simulink model "Robot_control"  (Simulink 8.0)
settings: Solver=ode45  SolverMode=SingleTasking  StartTime=0.0  StopTime=10  RelTol=1e-3
libraries: mblibv1 x4, vrlib x1
settings Model: Creator=zigg  LastModifiedBy=nakano  CovMetricSettings=dwe  CovHtmlReporting=off  covSaveCumulativeToWorkspaceVar=off  CovSaveSingleToWorkspaceVar=off  CovExternalEMLEnable=on
settings DataIOCC: LimitDataPoints=off  SaveFormat=StructureWithTime
settings OptimizationCC: ExpressionDepthLimit=128
settings DebuggingCC: UnderspecifiedInitializationDetection=Simplified  MergeDetectMultiDrivingBlocksExec=error  SolverPrmCheckMsg=none  FcnCallInpInsideContextMsg=EnableAllAsWarning  FrameProcessingCompatibilityMsg=error  StateNameClashWarn=none  SFUnexpectedBacktrackingDiag=error  SFNoUnconditionalDefaultTransitionDiag=error
settings HardwareCC: ProdBitPerPointer=64  ProdLargestAtomicFloat=Float  ProdIntDivRoundTo=Zero  ProdEndianess=LittleEndian  ProdHWDeviceType=Specified
settings ModelReferenceCC: PropagateSignalLabelsOutOfModel=on
settings CodeAppCC: CustomSymbolStrType=$N$R$M_T
settings GRTTargetCC: CodeReplacementLibrary=C99 (ISO)  GeneratePreprocessorConditionals=Use local settings

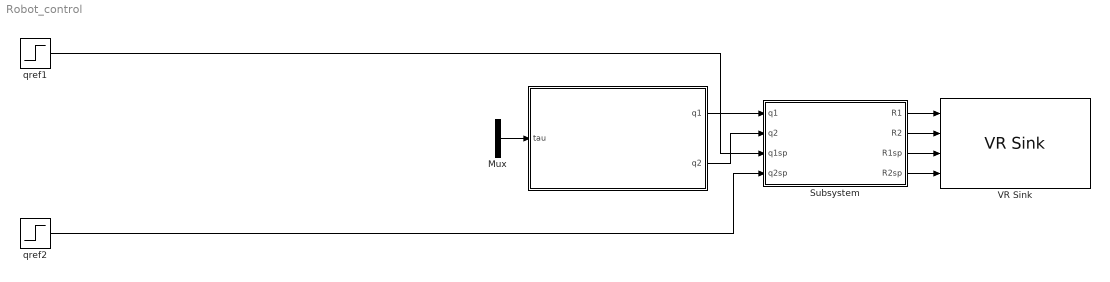
== system Robot_control ==
  "  " : Subsystem
  Mux : Mux  Inputs=2
  Subsystem : Subsystem
  VR Sink : vrlib/VR Sink  InstantiateOnLoad=on  SampleTime=0.1  ViewEnable=on  RemoteChange=off  RemoteView=off  FieldsWritten=Joint1.rotation.4.1.1.double#Joint2.rotation.4.1.1.double#Joint1_SP.rotation.4.1.1.double#Joint2_SP.rotation.4.1.1.double  WorldFileName=my_robot.wrl  AutoView=off  VideoDimensions=[]  AllowVariableSize=off
  qref1 : Step  SampleTime=0
  qref2 : Step  SampleTime=0
  wires:
  Subsystem/1(R1) -> VR Sink/1
  Subsystem/2(R2) -> VR Sink/2
  Subsystem/3(R1sp) -> VR Sink/3
  Subsystem/4(R2sp) -> VR Sink/4
  "  "/1(q1) -> Subsystem/1(q1)
  "  "/2(q2) -> Subsystem/2(q2)
  qref2/1 -> Subsystem/4(q2sp)
  qref1/1 -> Subsystem/3(q1sp)
  Mux/1 -> "  "/1(tau)

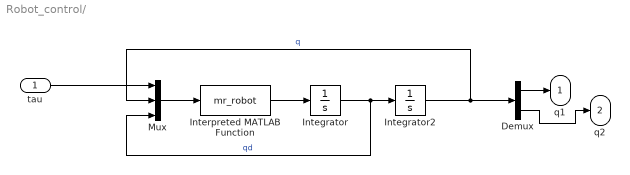
== system Robot_control/   ==
  tau : Inport
  Demux : Demux  Outputs=2
  Integrator : Integrator
  Integrator2 : Integrator  InitialCondition=pi/2*0
  Interpreted MATLAB Function : MATLABFcn  MATLABFcn=mr_robot  OutputDimensions=2
  Mux : Mux  Inputs=3
  q1 : Outport
  q2 : Outport  Port=2
  wires:
  Interpreted MATLAB Function/1 -> Integrator/1
  Integrator2/1 -> Demux/1, Mux/2  "q"
  Integrator/1 -> Mux/3, Integrator2/1  "qd"
  tau/1 -> Mux/1
  Mux/1 -> Interpreted MATLAB Function/1
  Demux/1 -> q1/1
  Demux/2 -> q2/1

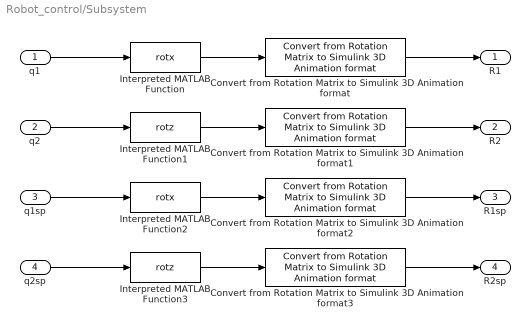
== system Robot_control/Subsystem ==
  q1 : Inport
  q2 : Inport  Port=2
  q1sp : Inport  Port=3
  q2sp : Inport  Port=4
  Convert from Rotation Matrix to Simulink 3D Animation format{,1..3} (4 alike) : mblibv1/Utilities/Convert from Rotation Matrix to Simulink 3D Animation format
  Interpreted MATLAB Function : MATLABFcn  MATLABFcn=rotx
  Interpreted MATLAB Function1 : MATLABFcn  MATLABFcn=rotz
  Interpreted MATLAB Function2 : MATLABFcn  MATLABFcn=rotx
  Interpreted MATLAB Function3 : MATLABFcn  MATLABFcn=rotz
  R1 : Outport
  R2 : Outport  Port=2
  R1sp : Outport  Port=3
  R2sp : Outport  Port=4
  wires:
  Convert from Rotation Matrix to Simulink 3D Animation format/1 -> R1/1
  Interpreted MATLAB Function/1 -> Convert from Rotation Matrix to Simulink 3D Animation format/1
  Interpreted MATLAB Function1/1 -> Convert from Rotation Matrix to Simulink 3D Animation format1/1
  Interpreted MATLAB Function2/1 -> Convert from Rotation Matrix to Simulink 3D Animation format2/1
  Interpreted MATLAB Function3/1 -> Convert from Rotation Matrix to Simulink 3D Animation format3/1
  q1/1 -> Interpreted MATLAB Function/1
  q2/1 -> Interpreted MATLAB Function1/1
  q1sp/1 -> Interpreted MATLAB Function2/1
  q2sp/1 -> Interpreted MATLAB Function3/1
  Convert from Rotation Matrix to Simulink 3D Animation format1/1 -> R2/1
  Convert from Rotation Matrix to Simulink 3D Animation format2/1 -> R1sp/1
  Convert from Rotation Matrix to Simulink 3D Animation format3/1 -> R2sp/1
